simulink model "four_to_one_MUX"  (R2021a)
settings: Solver=VariableStepAuto  StartTime=0.0  StopTime=10.0  RelTol=1e-3
settings Model: Creator=kbhar  LastModifiedBy=kbhar

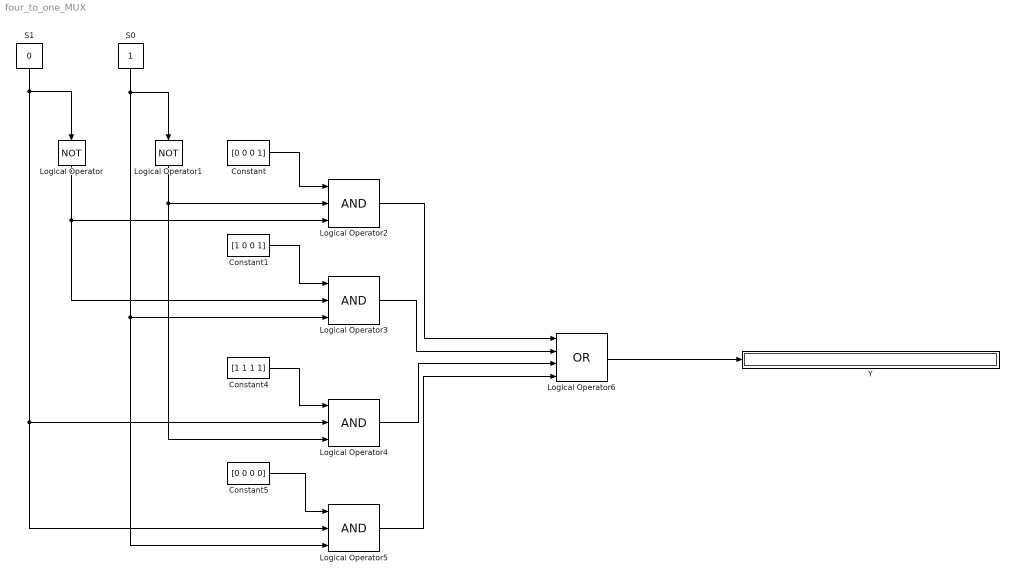
== system four_to_one_MUX ==
  Constant : Constant  Value=[0 0 0 1]
  Constant1 : Constant  Value=[1 0 0 1]
  Constant4 : Constant  Value=[1 1 1 1]
  Constant5 : Constant  Value=[0 0 0 0]
  Logical Operator : Logic  Operator=NOT  AllPortsSameDT=off  OutDataTypeStr=boolean
  Logical Operator1 : Logic  Operator=NOT  AllPortsSameDT=off  OutDataTypeStr=boolean
  Logical Operator{2..5} (4 alike) : Logic  Inputs=3  AllPortsSameDT=off  OutDataTypeStr=boolean
  Logical Operator6 : Logic  Operator=OR  Inputs=4  AllPortsSameDT=off  OutDataTypeStr=boolean
  S0 : Constant
  S1 : Constant  Value=0
  Y : Display
  wires:
  S1/1 -> Logical Operator4/2, Logical Operator5/2, Logical Operator/1
  S0/1 -> Logical Operator5/3, Logical Operator3/3, Logical Operator1/1
  Logical Operator/1 -> Logical Operator2/3, Logical Operator3/2
  Logical Operator1/1 -> Logical Operator2/2, Logical Operator4/3
  Constant1/1 -> Logical Operator3/1
  Logical Operator2/1 -> Logical Operator6/1
  Logical Operator3/1 -> Logical Operator6/2
  Logical Operator4/1 -> Logical Operator6/3
  Logical Operator5/1 -> Logical Operator6/4
  Logical Operator6/1 -> Y/1
  Constant/1 -> Logical Operator2/1
  Constant4/1 -> Logical Operator4/1
  Constant5/1 -> Logical Operator5/1
